simulink model "C28069_LLC_ePWM_V8_230307_PhaeShiftWorking"  (R2022b)
settings: Solver=FixedStepAuto  StartTime=0.0  StopTime=10  RelTol=1e-3  EnableMultiTasking=on
model workspace (MAT data in the model file):
  Comp_DAC = 512
undefined symbols (not defined in the file or in its folder): Down, GPTRIP1SEL, GPTRIP2SEL, PWM_Control, PWM_Gen, PWM_Gen1, SCI_A_Transmit, SCI_A_Transmit_Current_Suffix, SCI_A_Transmit_Duty_Suffix, SCI_A_Transmit_Freq_Suffix, SCI_A_Transmit_OVPFlag_Suffix, SCI_A_Transmit_PFC_Suffix, SCI_A_Transmit_SS_Suffix, SCI_A_Transmit_TBPHS_Suffix, SCI_A_Transmit_VADC_Suffix, SCI_A_Transmit_VAvg_Suffix, SCI_A_Transmit_VBAT_Suffix, SCI_A_Transmit_VBATRef_Suffix, SCI_A_Transmit_Vo_Suffix, TZ1, TZ2, u1, Up
libraries: c2802xlib x92, c280xlib x39, simulink x36, c2000lib x1
(part 14 of 18)

== system C28069_LLC_ePWM_V8_230307_PhaeShiftWorking/Softstart @5kHz/GetADC, FaultProtection, SoftStart  @5KHz/UpdatePWM/Frequency Update ==
  note: For Normal SoftStart
  note: For Reverse SoftStart
  function : TriggerPort  TriggerType=function-call  VariantControl=(inherit)
  Constant : Constant  Value=0  OutDataTypeStr=double
  Constant1 : Constant  Commented=on  Value=0
  Data Store Read : DataStoreRead  Commented=on  DataStoreName=Freq_Value  IndexOptions=Index vector (dialog)  Indices=1  OutputSizes=1
  Data Store Read1 : DataStoreRead  Commented=on  DataStoreName=PFC_OK  IndexOptions=Index vector (dialog)  Indices=1  OutputSizes=1
  Data Store Read10 : DataStoreRead  Commented=on  DataStoreName=OCP_Flag  IndexOptions=Index vector (dialog)  Indices=1  OutputSizes=1
  Data Store Read2 : DataStoreRead  Commented=on  DataStoreName=Duty_Value  IndexOptions=Index vector (dialog)  Indices=1  OutputSizes=1
  Data Store Read3 : DataStoreRead  DataStoreName=Freq_Value  IndexOptions=Index vector (dialog)  Indices=1  OutputSizes=1
  Data Store Read4 : DataStoreRead  DataStoreName=PFC_OK  IndexOptions=Index vector (dialog)  Indices=1  OutputSizes=1
  Data Store Read5 : DataStoreRead  Commented=on  DataStoreName=OVP_Flag  IndexOptions=Index vector (dialog)  Indices=1  OutputSizes=1
  Data Store Read6 : DataStoreRead  DataStoreName=OVP_Flag  IndexOptions=Index vector (dialog)  Indices=1  OutputSizes=1
  Data Store Read7 : DataStoreRead  DataStoreName=Freq_Value_Out  IndexOptions=Index vector (dialog)  Indices=1  OutputSizes=1
  Data Store Read8 : DataStoreRead  Commented=on  DataStoreName=Freq_Value_Out  IndexOptions=Index vector (dialog)  Indices=1  OutputSizes=1
  Data Store Read9 : DataStoreRead  DataStoreName=OCP_Flag  IndexOptions=Index vector (dialog)  Indices=1  OutputSizes=1
  Data Store Write : DataStoreWrite  DataStoreName=Freq_Value_Out  IndexOptions=Index vector (dialog)  Indices=1  OutputSizes=1
  Data Store Write1 : DataStoreWrite  Commented=on  DataStoreName=Freq_Value_Out  IndexOptions=Index vector (dialog)  Indices=1  OutputSizes=1
  Data Type Conversion : DataTypeConversion  Commented=on  OutDataTypeStr=uint16  SaturateOnIntegerOverflow=off  RndMeth=Floor
  Data Type Conversion3 : DataTypeConversion  Commented=on  OutDataTypeStr=uint16  SaturateOnIntegerOverflow=off  RndMeth=Floor
  Data Type Conversion4 : DataTypeConversion  Commented=on  OutDataTypeStr=uint16  SaturateOnIntegerOverflow=off  RndMeth=Floor
  Function Caller : FunctionCaller  Commented=on  FunctionPrototype=PWM_Gen1(u,u1)  InputArgumentSpecifications=<Enter example>  OutputArgumentSpecifications=<Enter example>
  Function Caller1 : FunctionCaller  FunctionPrototype=PWM_Gen(u)  InputArgumentSpecifications=<Enter example>  OutputArgumentSpecifications=<Enter example>
  Product : Product  Commented=on  Inputs=4  OutDataTypeStr=uint16
  Product1 : Product  Inputs=4  OutDataTypeStr=double
  Simulink Function1 : Subsystem  TreatAsAtomicUnit=on
  Simulink Function2 : Subsystem  Commented=on  TreatAsAtomicUnit=on
  Switch : Switch  Criteria=u2 > Threshold  OutDataTypeStr=double  SaturateOnIntegerOverflow=off  InputSameDT=off
  Switch1 : Switch  Commented=on  Criteria=u2 > Threshold  SaturateOnIntegerOverflow=off  InputSameDT=off
  wires:
  Data Store Read8/1 -> Data Type Conversion3/1
  Data Store Read3/1 -> Product1/1
  Data Type Conversion4/1 -> Function Caller/2
  Switch/1 -> Data Store Write/1
  Switch1/1 -> Data Store Write1/1
  Data Store Read6/1 -> Product1/3
  Data Type Conversion3/1 -> Function Caller/1
  Constant/1 -> Switch/3
  Data Store Read9/1 -> Product1/4
  Product/1 -> Switch1/1, Switch1/2
  Data Store Read/1 -> Product/1
  Data Store Read4/1 -> Product1/2
  Constant1/1 -> Switch1/3
  Data Store Read5/1 -> Product/3
  Data Store Read10/1 -> Product/4
  Data Store Read2/1 -> Data Type Conversion4/1
  Product1/1 -> Switch/1, Switch/2
  Data Store Read7/1 -> Function Caller1/1
  Data Type Conversion/1 -> Product/2
  Data Store Read1/1 -> Data Type Conversion/1

== system C28069_LLC_ePWM_V8_230307_PhaeShiftWorking/CloseLoop & Update @ ADCINT, 50kHz/Control/Frequency Update/Simulink Function1/Subsystem1 ==
  Frequency(kHz) : Inport  OutDataTypeStr=double
  Duty(%) : Inport  Port=2
  Constant1 : Constant  Value=90E6
  Divide : Product  Inputs=*/  RndMeth=Zero  SaturateOnIntegerOverflow=on
  Gain : Gain  Gain=1000
  Gain1 : Gain  Gain=1/100
  Gain2 : Gain  Gain=0.5
  Product : Product
  Product1 : Product
  Up-Down Counter : Constant  Value=2
  Out1 : Outport
  Out2 : Outport  Port=2
  Out3 : Outport  Port=3
  wires:
  Up-Down Counter/1 -> Product/2
  Gain/1 -> Product/1
  Product/1 -> Divide/2
  Frequency(kHz)/1 -> Gain/1
  Constant1/1 -> Divide/1
  Divide/1 -> Product1/1, Out1/1
  Duty(%)/1 -> Gain1/1
  Product1/1 -> Out2/1, Gain2/1
  Gain1/1 -> Product1/2
  Gain2/1 -> Out3/1

== system C28069_LLC_ePWM_V8_230307_PhaeShiftWorking/CloseLoop & Update @ ADCINT, 50kHz/Control/Frequency Update/Simulink Function2/Subsystem1 ==
  Frequency(kHz) : Inport
  Duty(%) : Inport  Port=2
  Constant1 : Constant  Value=90E6
  Divide : Product  Inputs=*/  RndMeth=Zero  SaturateOnIntegerOverflow=on
  Gain : Gain  Gain=1000
  Gain1 : Gain  Gain=1/100
  Gain2 : Gain  Gain=0.5
  Product : Product
  Product1 : Product
  Up-Down Counter : Constant  Value=2
  Out1 : Outport
  Out2 : Outport  Port=2
  Out3 : Outport  Port=3
  wires:
  Up-Down Counter/1 -> Product/2
  Gain/1 -> Product/1
  Product/1 -> Divide/2
  Frequency(kHz)/1 -> Gain/1
  Constant1/1 -> Divide/1
  Divide/1 -> Product1/1, Out1/1
  Duty(%)/1 -> Gain1/1
  Product1/1 -> Out2/1, Gain2/1
  Gain1/1 -> Product1/2
  Gain2/1 -> Out3/1

== system C28069_LLC_ePWM_V8_230307_PhaeShiftWorking/CloseLoop & Update @ ADCINT, 50kHz/Control/Frequency Update/Simulink Function3/Subsystem1 ==
  Frequency(kHz) : Inport  OutDataTypeStr=double
  Duty(%) : Inport  Port=2
  Constant1 : Constant  Value=90E6
  Divide : Product  Inputs=*/  RndMeth=Zero  SaturateOnIntegerOverflow=on
  Gain : Gain  Gain=1000
  Gain1 : Gain  Gain=1/100
  Gain2 : Gain  Gain=0.5
  Product : Product
  Product1 : Product
  Up-Down Counter : Constant  Value=2
  Out1 : Outport
  Out2 : Outport  Port=2
  Out3 : Outport  Port=3
  wires:
  Up-Down Counter/1 -> Product/2
  Gain/1 -> Product/1
  Product/1 -> Divide/2
  Frequency(kHz)/1 -> Gain/1
  Constant1/1 -> Divide/1
  Divide/1 -> Product1/1, Out1/1
  Duty(%)/1 -> Gain1/1
  Product1/1 -> Out2/1, Gain2/1
  Gain1/1 -> Product1/2
  Gain2/1 -> Out3/1

== system C28069_LLC_ePWM_V8_230307_PhaeShiftWorking/GetADC, FaultProtection, SoftStart  @5KHz/UpdatePWM/Frequency Update/Simulink Function1/Subsystem1 ==
  Frequency(kHz) : Inport  OutDataTypeStr=double
  Duty(%) : Inport  Port=2
  Constant1 : Constant  Value=90E6
  Divide : Product  Inputs=*/  RndMeth=Zero  SaturateOnIntegerOverflow=on
  Gain : Gain  Gain=1000
  Gain1 : Gain  Gain=1/100
  Gain2 : Gain  Gain=0.5
  Product : Product
  Product1 : Product
  Up-Down Counter : Constant  Value=2
  Out1 : Outport
  Out2 : Outport  Port=2
  Out3 : Outport  Port=3
  wires:
  Gain2/1 -> Out3/1
  Gain1/1 -> Product1/2
  Product1/1 -> Gain2/1, Out2/1
  Duty(%)/1 -> Gain1/1
  Divide/1 -> Out1/1, Product1/1
  Constant1/1 -> Divide/1
  Frequency(kHz)/1 -> Gain/1
  Product/1 -> Divide/2
  Gain/1 -> Product/1
  Up-Down Counter/1 -> Product/2

== system C28069_LLC_ePWM_V8_230307_PhaeShiftWorking/GetADC, FaultProtection, SoftStart  @5KHz/UpdatePWM/Frequency Update/Simulink Function2/Subsystem1 ==
  Frequency(kHz) : Inport
  Duty(%) : Inport  Port=2
  Constant1 : Constant  Value=90E6
  Divide : Product  Inputs=*/  RndMeth=Zero  SaturateOnIntegerOverflow=on
  Gain : Gain  Gain=1000
  Gain1 : Gain  Gain=1/100
  Gain2 : Gain  Gain=0.5
  Product : Product
  Product1 : Product
  Up-Down Counter : Constant  Value=2
  Out1 : Outport
  Out2 : Outport  Port=2
  Out3 : Outport  Port=3
  wires:
  Gain2/1 -> Out3/1
  Gain1/1 -> Product1/2
  Product1/1 -> Gain2/1, Out2/1
  Duty(%)/1 -> Gain1/1
  Divide/1 -> Out1/1, Product1/1
  Constant1/1 -> Divide/1
  Frequency(kHz)/1 -> Gain/1
  Product/1 -> Divide/2
  Gain/1 -> Product/1
  Up-Down Counter/1 -> Product/2

== system C28069_LLC_ePWM_V8_230307_PhaeShiftWorking/GetADC, FaultProtection, SoftStart  @5KHz/UpdatePWM1/Frequency Update/Simulink Function1/Subsystem1 ==
  Frequency(kHz) : Inport  OutDataTypeStr=double
  Duty(%) : Inport  Port=2
  Constant1 : Constant  Value=90E6
  Divide : Product  Inputs=*/  RndMeth=Zero  SaturateOnIntegerOverflow=on
  Gain : Gain  Gain=1000
  Gain1 : Gain  Gain=1/100
  Gain2 : Gain  Gain=0.5
  Product : Product
  Product1 : Product
  Up-Down Counter : Constant  Value=2
  Out1 : Outport
  Out2 : Outport  Port=2
  Out3 : Outport  Port=3
  wires:
  Up-Down Counter/1 -> Product/2
  Gain/1 -> Product/1
  Product/1 -> Divide/2
  Frequency(kHz)/1 -> Gain/1
  Constant1/1 -> Divide/1
  Divide/1 -> Product1/1, Out1/1
  Duty(%)/1 -> Gain1/1
  Product1/1 -> Out2/1, Gain2/1
  Gain1/1 -> Product1/2
  Gain2/1 -> Out3/1

== system C28069_LLC_ePWM_V8_230307_PhaeShiftWorking/GetADC, FaultProtection, SoftStart  @5KHz/UpdatePWM1/Frequency Update/Simulink Function2/Subsystem1 ==
  Frequency(kHz) : Inport
  Duty(%) : Inport  Port=2
  Constant1 : Constant  Value=90E6
  Divide : Product  Inputs=*/  RndMeth=Zero  SaturateOnIntegerOverflow=on
  Gain : Gain  Gain=1000
  Gain1 : Gain  Gain=1/100
  Gain2 : Gain  Gain=0.5
  Product : Product
  Product1 : Product
  Up-Down Counter : Constant  Value=2
  Out1 : Outport
  Out2 : Outport  Port=2
  Out3 : Outport  Port=3
  wires:
  Up-Down Counter/1 -> Product/2
  Gain/1 -> Product/1
  Product/1 -> Divide/2
  Frequency(kHz)/1 -> Gain/1
  Constant1/1 -> Divide/1
  Divide/1 -> Product1/1, Out1/1
  Duty(%)/1 -> Gain1/1
  Product1/1 -> Out2/1, Gain2/1
  Gain1/1 -> Product1/2
  Gain2/1 -> Out3/1

== system C28069_LLC_ePWM_V8_230307_PhaeShiftWorking/GetADC, FaultProtection, SoftStart  @5KHz/UpdatePWM1/Frequency Update/Simulink Function3/Subsystem1 ==
  Frequency(kHz) : Inport  OutDataTypeStr=double
  Duty(%) : Inport  Port=2
  Constant1 : Constant  Value=90E6
  Divide : Product  Inputs=*/  RndMeth=Zero  SaturateOnIntegerOverflow=on
  Gain : Gain  Gain=1000
  Gain1 : Gain  Gain=1/100
  Gain2 : Gain  Gain=0.5
  Product : Product
  Product1 : Product
  Up-Down Counter : Constant  Value=2
  Out1 : Outport
  Out2 : Outport  Port=2
  Out3 : Outport  Port=3
  wires:
  Up-Down Counter/1 -> Product/2
  Gain/1 -> Product/1
  Product/1 -> Divide/2
  Frequency(kHz)/1 -> Gain/1
  Constant1/1 -> Divide/1
  Divide/1 -> Product1/1, Out1/1
  Duty(%)/1 -> Gain1/1
  Product1/1 -> Out2/1, Gain2/1
  Gain1/1 -> Product1/2
  Gain2/1 -> Out3/1

== system C28069_LLC_ePWM_V8_230307_PhaeShiftWorking/GetADC, FaultProtection, SoftStart  @5KHz/UpdatePWM1/SoftStart/If Action Subsystem/ReservseSoftStart1 ==
  function : TriggerPort  TriggerType=function-call  VariantControl=(inherit)
  Chart1 : Stateflow chart  TreatAsAtomicUnit=on
  Constant : Constant  Value=160  OutDataTypeStr=double  SampleTime=Inf
  Constant1 : Constant  Value=200  OutDataTypeStr=double  SampleTime=Inf
  Constant2 : Constant  SampleTime=Inf
  Data Store Read : DataStoreRead  DataStoreName=PFC_OK  IndexOptions=Index vector (dialog)  Indices=1  OutputSizes=1
  Data Store Write1 : DataStoreWrite  DataStoreName=SoftStart_OK_Signal  IndexOptions=Index vector (dialog)  Indices=1  OutputSizes=1
  Data Store Write2 : DataStoreWrite  DataStoreName=Freq_Value  IndexOptions=Index vector (dialog)  Indices=1  OutputSizes=1
  Data Store Write3 : DataStoreWrite  DataStoreName=Duty_Value  IndexOptions=Index vector (dialog)  Indices=1  OutputSizes=1
  Data Type Conversion : DataTypeConversion  OutDataTypeStr=uint16  SaturateOnIntegerOverflow=off  RndMeth=Floor
  Data Type Conversion1 : DataTypeConversion  OutDataTypeStr=uint16  SaturateOnIntegerOverflow=off  RndMeth=Floor
  Data Type Conversion2 : DataTypeConversion  Commented=on  OutDataTypeStr=uint8  SaturateOnIntegerOverflow=off  RndMeth=Floor
  ms : Constant  Commented=on  Value=15  SampleTime=Inf
  wires:
  Constant1/1 -> Chart1/3(Resonant_Frequency)
  Constant/1 -> Chart1/2(Initial_Frequency)
  Data Type Conversion/1 -> Data Store Write2/1
  Chart1/3(Frequency_Adjusted) -> Data Type Conversion/1
  Chart1/1(SoftStart_OK) -> Data Store Write1/1
  Chart1/2(Duty_Adjusted) -> Data Type Conversion1/1
  Data Type Conversion1/1 -> Data Store Write3/1
  Data Store Read/1 -> Chart1/1(PFC_OK)

== system C28069_LLC_ePWM_V8_230307_PhaeShiftWorking/GetADC, FaultProtection, SoftStart  @5KHz/UpdatePWM1/SoftStart/If Action Subsystem/SoftStart1 ==
  function : TriggerPort  TriggerType=function-call  VariantControl=(inherit)
  Chart : Stateflow chart  TreatAsAtomicUnit=on
  Chart1 : Stateflow chart  Commented=on  TreatAsAtomicUnit=on
  Constant : Constant  Commented=on  Value=153  OutDataTypeStr=double  SampleTime=Inf
  Constant1 : Constant  Commented=on  Value=130  OutDataTypeStr=double  SampleTime=Inf
  Constant2 : Constant  Value=15  OutDataTypeStr=double  SampleTime=Inf
  Data Store Read : DataStoreRead  Commented=on  DataStoreName=PFC_OK  IndexOptions=Index vector (dialog)  Indices=1  OutputSizes=1
  Data Store Read1 : DataStoreRead  DataStoreName=PFC_OK  IndexOptions=Index vector (dialog)  Indices=1  OutputSizes=1
  Data Store Read2 : DataStoreRead  DataStoreName=VBAT_Value  IndexOptions=Index vector (dialog)  Indices=1  OutputSizes=1
  Data Store Write : DataStoreWrite  DataStoreName=VBAT_Ref_Value  IndexOptions=Index vector (dialog)  Indices=1  OutputSizes=1
  Data Store Write1 : DataStoreWrite  Commented=on  DataStoreName=SoftStart_OK_Signal  IndexOptions=Index vector (dialog)  Indices=1  OutputSizes=1
  Data Store Write2 : DataStoreWrite  Commented=on  DataStoreName=Freq_Value  IndexOptions=Index vector (dialog)  Indices=1  OutputSizes=1
  Data Store Write3 : DataStoreWrite  DataStoreName=SoftStart_OK_Signal  IndexOptions=Index vector (dialog)  Indices=1  OutputSizes=1
  GPIO21 : c280xlib/Digital Output  GPIO_Number=GPIO16~GPIO23  GPIO_Bit0=off  GPIO_BIT0_Toggle=off  GPIO_Bit1=off  GPIO_BIT1_Toggle=off  GPIO_Bit2=off  GPIO_BIT2_Toggle=off  GPIO_Bit3=off  GPIO_BIT3_Toggle=off  GPIO_Bit4=off  GPIO_BIT4_Toggle=off  GPIO_Bit5=on  GPIO_BIT5_Toggle=off  GPIO_Bit6=off  GPIO_BIT6_Toggle=off  GPIO_Bit7=off  GPIO_BIT7_Toggle=off
  wires:
  Chart1/1(SoftStart_OK) -> Data Store Write1/1
  Chart1/2(Frequency_Adjusted) -> Data Store Write2/1
  Constant/1 -> Chart1/2(Initial_Frequency)
  Constant1/1 -> Chart1/3(Resonant_Frequency)
  Data Store Read/1 -> Chart1/1(PFC_OK)
  Data Store Read1/1 -> GPIO21/1, Chart/1(PFC_OK)
  Constant2/1 -> Chart/3(VBAT_Ref)
  Data Store Read2/1 -> Chart/2(VBAT_Value)
  Chart/1(VBAT_Ref_adjusted) -> Data Store Write/1
  Chart/2(SoftStart_OK) -> Data Store Write3/1

== system C28069_LLC_ePWM_V8_230307_PhaeShiftWorking/Softstart @5kHz/GetADC, FaultProtection, SoftStart  @5KHz/Fault Protection @ 5KHz/If Action Subsystem/OCP ==
  note: 1900 = @>1.9A Load will trigger
  note: False
  note: Average the value
  note: True
  function : TriggerPort  TriggerType=function-call  VariantControl=(inherit)
  ADC : c2802xlib/ADC  Commented=on  blkParamProc=C2000  ADCModule=1  samplingMode=Single sample mode  ADCResolution=12-bit (Single-ended input)  useSOC1=SOC0  useSOC2=SOC0_SOC1  SOCAcquisitionWindow=7  SOCTriggerSource=ePWM5_ADCSOCA  SOCInterruptTrigger=No ADCINT  Ts=-1  dType=uint16  postInterrupt=off  interruptSel=ADCINT1  ADCINTContinuous=off  endma=off  chdma=1  conv1=ADCINA2  conv2=ADCINA0 and ADCINB0  conv1_Type4=ADCIN0  conv2_Type4=ADCIN0 and ADCIN1
      settings: LibrarySourceBlock=c2806xlib/ADC
  Constant3 : Constant  Value=0  OutDataTypeStr=single
  Data Store Read : DataStoreRead  DataStoreName=OCP_Flag  IndexOptions=Index vector (dialog)  Indices=1  OutputSizes=1
  Data Store Read1 : DataStoreRead  DataStoreName=IoutCurrentBAT_Value  IndexOptions=Index vector (dialog)  Indices=1  OutputSizes=1
  Data Store Write2 : DataStoreWrite  DataStoreName=OCP_Flag  IndexOptions=Index vector (dialog)  Indices=1  OutputSizes=1
  Data Type Conversion1 : DataTypeConversion  OutDataTypeStr=double  SaturateOnIntegerOverflow=off  RndMeth=Floor
  Delay : Delay  Commented=on  DelayLength=1
  Delay1 : Delay  Commented=on
  Delay2 : Delay  Commented=on  DelayLength=3
  Delay3 : Delay  Commented=on  DelayLength=4
  Delay4 : Delay  Commented=on  DelayLength=5
  Display7 : Display
  Gain : Gain  Commented=on  Gain=1/6  OutDataTypeStr=uint16
  Sum : Sum  Commented=on  Inputs=|++++++
  Switch : Switch  Criteria=u2 > Threshold  Threshold=2100  OutDataTypeStr=single  SaturateOnIntegerOverflow=off  InputSameDT=off
  wires:
  Data Store Read1/1 -> Switch/2, Display7/1
  Delay4/1 -> Sum/6
  Delay3/1 -> Sum/5
  Gain/1 -> Delay/1, Delay1/1, Delay2/1, Delay3/1, Delay4/1
  Delay/1 -> Sum/2
  Delay1/1 -> Sum/3
  Delay2/1 -> Sum/4
  Sum/1 -> Gain/1
  Data Type Conversion1/1 -> Data Store Write2/1
  Data Store Read/1 -> Switch/3
  Constant3/1 -> Switch/1
  Switch/1 -> Data Type Conversion1/1
  ADC/1 -> Sum/1

== system C28069_LLC_ePWM_V8_230307_PhaeShiftWorking/Softstart @5kHz/GetADC, FaultProtection, SoftStart  @5KHz/Fault Protection @ 5KHz/If Action Subsystem/OVP ==
  note: True
  note: Average the value
  note: False
  note: >92Vdc will trigger
  function : TriggerPort  TriggerType=function-call  VariantControl=(inherit)
  ADC : c2802xlib/ADC  Commented=on  blkParamProc=C2000  ADCModule=1  samplingMode=Single sample mode  ADCResolution=12-bit (Single-ended input)  useSOC1=SOC0  useSOC2=SOC0_SOC1  SOCAcquisitionWindow=7  SOCTriggerSource=ePWM5_ADCSOCA  SOCInterruptTrigger=No ADCINT  Ts=-1  dType=uint16  postInterrupt=off  interruptSel=ADCINT1  ADCINTContinuous=off  endma=off  chdma=1  conv1=ADCINA2  conv2=ADCINA0 and ADCINB0  conv1_Type4=ADCIN0  conv2_Type4=ADCIN0 and ADCIN1
      settings: LibrarySourceBlock=c2806xlib/ADC
  Constant3 : Constant  Value=0  OutDataTypeStr=single
  Data Store Read : DataStoreRead  DataStoreName=OVP_Flag  IndexOptions=Index vector (dialog)  Indices=1  OutputSizes=1
  Data Store Read1 : DataStoreRead  DataStoreName=VBAT_Value  IndexOptions=Index vector (dialog)  Indices=1  OutputSizes=1
  Data Store Write2 : DataStoreWrite  DataStoreName=OVP_Flag  IndexOptions=Index vector (dialog)  Indices=1  OutputSizes=1
  Data Type Conversion1 : DataTypeConversion  OutDataTypeStr=double  SaturateOnIntegerOverflow=off  RndMeth=Floor
  Delay : Delay  Commented=on  DelayLength=1
  Delay1 : Delay  Commented=on
  Delay2 : Delay  Commented=on  DelayLength=3
  Delay3 : Delay  Commented=on  DelayLength=4
  Delay4 : Delay  Commented=on  DelayLength=5
  Display7 : Display
  Gain : Gain  Commented=on  Gain=1/6  OutDataTypeStr=uint16
  Sum : Sum  Commented=on  Inputs=|++++++
  Switch : Switch  Criteria=u2 > Threshold  Threshold=35  OutDataTypeStr=single  SaturateOnIntegerOverflow=off  InputSameDT=off
  wires:
  ADC/1 -> Sum/1
  Switch/1 -> Data Type Conversion1/1
  Constant3/1 -> Switch/1
  Data Store Read/1 -> Switch/3
  Data Type Conversion1/1 -> Data Store Write2/1
  Sum/1 -> Gain/1
  Delay2/1 -> Sum/4
  Delay1/1 -> Sum/3
  Delay/1 -> Sum/2
  Gain/1 -> Delay4/1, Delay3/1, Delay2/1, Delay1/1, Delay/1
  Delay3/1 -> Sum/5
  Delay4/1 -> Sum/6
  Data Store Read1/1 -> Display7/1, Switch/2

== system C28069_LLC_ePWM_V8_230307_PhaeShiftWorking/Softstart @5kHz/GetADC, FaultProtection, SoftStart  @5KHz/Fault Protection @ 5KHz/If Action Subsystem/TestToCheckOVPFlag ==
  note: Comment out GPIO14 when flash to MB, as SCI_B using GPIO14
  note: Test to check if this OVP_Flag is working
  function : TriggerPort  TriggerType=function-call  VariantControl=(inherit)
  Data Store Read : DataStoreRead  DataStoreName=OVP_Flag  IndexOptions=Index vector (dialog)  Indices=1  OutputSizes=1
  GPIO14 Test : c280xlib/Digital Output  GPIO_Number=GPIO8~GPIO15  GPIO_Bit0=off  GPIO_BIT0_Toggle=off  GPIO_Bit1=off  GPIO_BIT1_Toggle=off  GPIO_Bit2=off  GPIO_BIT2_Toggle=off  GPIO_Bit3=off  GPIO_BIT3_Toggle=off  GPIO_Bit4=off  GPIO_BIT4_Toggle=off  GPIO_Bit5=off  GPIO_BIT5_Toggle=off  GPIO_Bit6=on  GPIO_BIT6_Toggle=off  GPIO_Bit7=off  GPIO_BIT7_Toggle=off
  wires:
  Data Store Read/1 -> GPIO14 Test/1

== system C28069_LLC_ePWM_V8_230307_PhaeShiftWorking/Softstart @5kHz/GetADC, FaultProtection, SoftStart  @5KHz/Fault Protection @ 5KHz1/If Action Subsystem/OCP ==
  note: 1900 = @>1.9A Load will trigger
  note: False
  note: Average the value
  note: True
  function : TriggerPort  TriggerType=function-call  VariantControl=(inherit)
  ADC : c2802xlib/ADC  Commented=on  blkParamProc=C2000  ADCModule=1  samplingMode=Single sample mode  ADCResolution=12-bit (Single-ended input)  useSOC1=SOC0  useSOC2=SOC0_SOC1  SOCAcquisitionWindow=7  SOCTriggerSource=ePWM5_ADCSOCA  SOCInterruptTrigger=No ADCINT  Ts=-1  dType=uint16  postInterrupt=off  interruptSel=ADCINT1  ADCINTContinuous=off  endma=off  chdma=1  conv1=ADCINA2  conv2=ADCINA0 and ADCINB0  conv1_Type4=ADCIN0  conv2_Type4=ADCIN0 and ADCIN1
      settings: LibrarySourceBlock=c2806xlib/ADC
  Constant3 : Constant  Value=0  OutDataTypeStr=single
  Data Store Read : DataStoreRead  DataStoreName=OCP_Flag  IndexOptions=Index vector (dialog)  Indices=1  OutputSizes=1
  Data Store Read1 : DataStoreRead  DataStoreName=IoutCurrentBAT_Value  IndexOptions=Index vector (dialog)  Indices=1  OutputSizes=1
  Data Store Write2 : DataStoreWrite  DataStoreName=OCP_Flag  IndexOptions=Index vector (dialog)  Indices=1  OutputSizes=1
  Data Type Conversion1 : DataTypeConversion  OutDataTypeStr=double  SaturateOnIntegerOverflow=off  RndMeth=Floor
  Delay : Delay  Commented=on  DelayLength=1
  Delay1 : Delay  Commented=on
  Delay2 : Delay  Commented=on  DelayLength=3
  Delay3 : Delay  Commented=on  DelayLength=4
  Delay4 : Delay  Commented=on  DelayLength=5
  Display7 : Display
  Gain : Gain  Commented=on  Gain=1/6  OutDataTypeStr=uint16
  Sum : Sum  Commented=on  Inputs=|++++++
  Switch : Switch  Criteria=u2 > Threshold  Threshold=2100  OutDataTypeStr=single  SaturateOnIntegerOverflow=off  InputSameDT=off
  wires:
  Data Store Read1/1 -> Switch/2, Display7/1
  Delay4/1 -> Sum/6
  Delay3/1 -> Sum/5
  Gain/1 -> Delay/1, Delay1/1, Delay2/1, Delay3/1, Delay4/1
  Delay/1 -> Sum/2
  Delay1/1 -> Sum/3
  Delay2/1 -> Sum/4
  Sum/1 -> Gain/1
  Data Type Conversion1/1 -> Data Store Write2/1
  Data Store Read/1 -> Switch/3
  Constant3/1 -> Switch/1
  Switch/1 -> Data Type Conversion1/1
  ADC/1 -> Sum/1

== system C28069_LLC_ePWM_V8_230307_PhaeShiftWorking/Softstart @5kHz/GetADC, FaultProtection, SoftStart  @5KHz/Fault Protection @ 5KHz1/If Action Subsystem/OVP ==
  note: True
  note: Average the value
  note: False
  note: >92Vdc will trigger
  function : TriggerPort  TriggerType=function-call  VariantControl=(inherit)
  ADC : c2802xlib/ADC  Commented=on  blkParamProc=C2000  ADCModule=1  samplingMode=Single sample mode  ADCResolution=12-bit (Single-ended input)  useSOC1=SOC0  useSOC2=SOC0_SOC1  SOCAcquisitionWindow=7  SOCTriggerSource=ePWM5_ADCSOCA  SOCInterruptTrigger=No ADCINT  Ts=-1  dType=uint16  postInterrupt=off  interruptSel=ADCINT1  ADCINTContinuous=off  endma=off  chdma=1  conv1=ADCINA2  conv2=ADCINA0 and ADCINB0  conv1_Type4=ADCIN0  conv2_Type4=ADCIN0 and ADCIN1
      settings: LibrarySourceBlock=c2806xlib/ADC
  Constant3 : Constant  Value=0  OutDataTypeStr=single
  Data Store Read : DataStoreRead  DataStoreName=OVP_Flag  IndexOptions=Index vector (dialog)  Indices=1  OutputSizes=1
  Data Store Read1 : DataStoreRead  DataStoreName=VBAT_Value  IndexOptions=Index vector (dialog)  Indices=1  OutputSizes=1
  Data Store Write2 : DataStoreWrite  DataStoreName=OVP_Flag  IndexOptions=Index vector (dialog)  Indices=1  OutputSizes=1
  Data Type Conversion1 : DataTypeConversion  OutDataTypeStr=double  SaturateOnIntegerOverflow=off  RndMeth=Floor
  Delay : Delay  Commented=on  DelayLength=1
  Delay1 : Delay  Commented=on
  Delay2 : Delay  Commented=on  DelayLength=3
  Delay3 : Delay  Commented=on  DelayLength=4
  Delay4 : Delay  Commented=on  DelayLength=5
  Display7 : Display
  Gain : Gain  Commented=on  Gain=1/6  OutDataTypeStr=uint16
  Sum : Sum  Commented=on  Inputs=|++++++
  Switch : Switch  Criteria=u2 > Threshold  Threshold=35  OutDataTypeStr=single  SaturateOnIntegerOverflow=off  InputSameDT=off
  wires:
  ADC/1 -> Sum/1
  Switch/1 -> Data Type Conversion1/1
  Constant3/1 -> Switch/1
  Data Store Read/1 -> Switch/3
  Data Type Conversion1/1 -> Data Store Write2/1
  Sum/1 -> Gain/1
  Delay2/1 -> Sum/4
  Delay1/1 -> Sum/3
  Delay/1 -> Sum/2
  Gain/1 -> Delay4/1, Delay3/1, Delay2/1, Delay1/1, Delay/1
  Delay3/1 -> Sum/5
  Delay4/1 -> Sum/6
  Data Store Read1/1 -> Display7/1, Switch/2

== system C28069_LLC_ePWM_V8_230307_PhaeShiftWorking/Softstart @5kHz/GetADC, FaultProtection, SoftStart  @5KHz/Fault Protection @ 5KHz1/If Action Subsystem/TestToCheckOVPFlag ==
  note: Comment out GPIO14 when flash to MB, as SCI_B using GPIO14
  note: Test to check if this OVP_Flag is working
  function : TriggerPort  TriggerType=function-call  VariantControl=(inherit)
  Data Store Read : DataStoreRead  DataStoreName=OVP_Flag  IndexOptions=Index vector (dialog)  Indices=1  OutputSizes=1
  GPIO14 Test : c280xlib/Digital Output  GPIO_Number=GPIO8~GPIO15  GPIO_Bit0=off  GPIO_BIT0_Toggle=off  GPIO_Bit1=off  GPIO_BIT1_Toggle=off  GPIO_Bit2=off  GPIO_BIT2_Toggle=off  GPIO_Bit3=off  GPIO_BIT3_Toggle=off  GPIO_Bit4=off  GPIO_BIT4_Toggle=off  GPIO_Bit5=off  GPIO_BIT5_Toggle=off  GPIO_Bit6=on  GPIO_BIT6_Toggle=off  GPIO_Bit7=off  GPIO_BIT7_Toggle=off
  wires:
  Data Store Read/1 -> GPIO14 Test/1

== system C28069_LLC_ePWM_V8_230307_PhaeShiftWorking/Softstart @5kHz/GetADC, FaultProtection, SoftStart  @5KHz/Frequency Update/Simulink Function1/Subsystem1 ==
  Frequency(kHz) : Inport  OutDataTypeStr=double
  Duty(%) : Inport  Port=2
  Constant1 : Constant  Value=90E6
  Divide : Product  Inputs=*/  RndMeth=Zero  SaturateOnIntegerOverflow=on
  Gain : Gain  Gain=1000
  Gain1 : Gain  Gain=1/100
  Gain2 : Gain  Gain=0.5
  Product : Product
  Product1 : Product
  Up-Down Counter : Constant  Value=2
  Out1 : Outport
  Out2 : Outport  Port=2
  Out3 : Outport  Port=3
  wires:
  Up-Down Counter/1 -> Product/2
  Gain/1 -> Product/1
  Product/1 -> Divide/2
  Frequency(kHz)/1 -> Gain/1
  Constant1/1 -> Divide/1
  Divide/1 -> Product1/1, Out1/1
  Duty(%)/1 -> Gain1/1
  Product1/1 -> Out2/1, Gain2/1
  Gain1/1 -> Product1/2
  Gain2/1 -> Out3/1

== system C28069_LLC_ePWM_V8_230307_PhaeShiftWorking/Softstart @5kHz/GetADC, FaultProtection, SoftStart  @5KHz/Frequency Update/Simulink Function2/Subsystem1 ==
  Frequency(kHz) : Inport
  Duty(%) : Inport  Port=2
  Constant1 : Constant  Value=90E6
  Divide : Product  Inputs=*/  RndMeth=Zero  SaturateOnIntegerOverflow=on
  Gain : Gain  Gain=1000
  Gain1 : Gain  Gain=1/100
  Gain2 : Gain  Gain=0.5
  Product : Product
  Product1 : Product
  Up-Down Counter : Constant  Value=2
  Out1 : Outport
  Out2 : Outport  Port=2
  Out3 : Outport  Port=3
  wires:
  Up-Down Counter/1 -> Product/2
  Gain/1 -> Product/1
  Product/1 -> Divide/2
  Frequency(kHz)/1 -> Gain/1
  Constant1/1 -> Divide/1
  Divide/1 -> Product1/1, Out1/1
  Duty(%)/1 -> Gain1/1
  Product1/1 -> Out2/1, Gain2/1
  Gain1/1 -> Product1/2
  Gain2/1 -> Out3/1

== system C28069_LLC_ePWM_V8_230307_PhaeShiftWorking/Softstart @5kHz/GetADC, FaultProtection, SoftStart  @5KHz/Frequency Update/Simulink Function3/Subsystem1 ==
  Frequency(kHz) : Inport  OutDataTypeStr=double
  Duty(%) : Inport  Port=2
  Constant1 : Constant  Value=90E6
  Divide : Product  Inputs=*/  RndMeth=Zero  SaturateOnIntegerOverflow=on
  Gain : Gain  Gain=1000
  Gain1 : Gain  Gain=1/100
  Gain2 : Gain  Gain=0.5
  Product : Product
  Product1 : Product
  Up-Down Counter : Constant  Value=2
  Out1 : Outport
  Out2 : Outport  Port=2
  Out3 : Outport  Port=3
  wires:
  Up-Down Counter/1 -> Product/2
  Gain/1 -> Product/1
  Product/1 -> Divide/2
  Frequency(kHz)/1 -> Gain/1
  Constant1/1 -> Divide/1
  Divide/1 -> Product1/1, Out1/1
  Duty(%)/1 -> Gain1/1
  Product1/1 -> Out2/1, Gain2/1
  Gain1/1 -> Product1/2
  Gain2/1 -> Out3/1

== system C28069_LLC_ePWM_V8_230307_PhaeShiftWorking/Softstart @5kHz/GetADC, FaultProtection, SoftStart  @5KHz/SoftStart/If Action Subsystem/ReservseSoftStart ==
  function : TriggerPort  TriggerType=function-call  VariantControl=(inherit)
  Chart1 : Stateflow chart  TreatAsAtomicUnit=on
  Constant : Constant  Value=160  OutDataTypeStr=double  SampleTime=Inf
  Constant1 : Constant  Value=200  OutDataTypeStr=double  SampleTime=Inf
  Constant2 : Constant  SampleTime=Inf
  Data Store Read : DataStoreRead  DataStoreName=PFC_OK  IndexOptions=Index vector (dialog)  Indices=1  OutputSizes=1
  Data Store Write1 : DataStoreWrite  DataStoreName=SoftStart_OK_Signal  IndexOptions=Index vector (dialog)  Indices=1  OutputSizes=1
  Data Store Write2 : DataStoreWrite  DataStoreName=Freq_Value  IndexOptions=Index vector (dialog)  Indices=1  OutputSizes=1
  Data Store Write3 : DataStoreWrite  DataStoreName=Duty_Value  IndexOptions=Index vector (dialog)  Indices=1  OutputSizes=1
  Data Type Conversion : DataTypeConversion  OutDataTypeStr=uint16  SaturateOnIntegerOverflow=off  RndMeth=Floor
  Data Type Conversion1 : DataTypeConversion  OutDataTypeStr=uint16  SaturateOnIntegerOverflow=off  RndMeth=Floor
  Data Type Conversion2 : DataTypeConversion  Commented=on  OutDataTypeStr=uint8  SaturateOnIntegerOverflow=off  RndMeth=Floor
  ms : Constant  Commented=on  Value=15  SampleTime=Inf
  wires:
  Constant1/1 -> Chart1/3(Resonant_Frequency)
  Constant/1 -> Chart1/2(Initial_Frequency)
  Data Type Conversion/1 -> Data Store Write2/1
  Chart1/3(Frequency_Adjusted) -> Data Type Conversion/1
  Chart1/1(SoftStart_OK) -> Data Store Write1/1
  Chart1/2(Duty_Adjusted) -> Data Type Conversion1/1
  Data Type Conversion1/1 -> Data Store Write3/1
  Data Store Read/1 -> Chart1/1(PFC_OK)

== system C28069_LLC_ePWM_V8_230307_PhaeShiftWorking/Softstart @5kHz/GetADC, FaultProtection, SoftStart  @5KHz/SoftStart/If Action Subsystem/SoftStart ==
  function : TriggerPort  TriggerType=function-call  VariantControl=(inherit)
  Chart1 : Stateflow chart  TreatAsAtomicUnit=on
  Constant : Constant  Value=153  OutDataTypeStr=double  SampleTime=Inf
  Constant1 : Constant  Value=130  OutDataTypeStr=double  SampleTime=Inf
  Data Store Read : DataStoreRead  DataStoreName=PFC_OK  IndexOptions=Index vector (dialog)  Indices=1  OutputSizes=1
  Data Store Write1 : DataStoreWrite  DataStoreName=SoftStart_OK_Signal  IndexOptions=Index vector (dialog)  Indices=1  OutputSizes=1
  Data Store Write2 : DataStoreWrite  DataStoreName=Freq_Value  IndexOptions=Index vector (dialog)  Indices=1  OutputSizes=1
  wires:
  Chart1/1(SoftStart_OK) -> Data Store Write1/1
  Chart1/2(Frequency_Adjusted) -> Data Store Write2/1
  Constant/1 -> Chart1/2(Initial_Frequency)
  Constant1/1 -> Chart1/3(Resonant_Frequency)
  Data Store Read/1 -> Chart1/1(PFC_OK)

== system C28069_LLC_ePWM_V8_230307_PhaeShiftWorking/Softstart @5kHz/GetADC, FaultProtection, SoftStart  @5KHz/SoftStart1/If Action Subsystem/ReservseSoftStart1 ==
  function : TriggerPort  TriggerType=function-call  VariantControl=(inherit)
  Chart1 : Stateflow chart  TreatAsAtomicUnit=on
  Constant : Constant  Value=160  OutDataTypeStr=double  SampleTime=Inf
  Constant1 : Constant  Value=200  OutDataTypeStr=double  SampleTime=Inf
  Constant2 : Constant  SampleTime=Inf
  Data Store Read : DataStoreRead  DataStoreName=PFC_OK  IndexOptions=Index vector (dialog)  Indices=1  OutputSizes=1
  Data Store Write1 : DataStoreWrite  DataStoreName=SoftStart_OK_Signal  IndexOptions=Index vector (dialog)  Indices=1  OutputSizes=1
  Data Store Write2 : DataStoreWrite  DataStoreName=Freq_Value  IndexOptions=Index vector (dialog)  Indices=1  OutputSizes=1
  Data Store Write3 : DataStoreWrite  DataStoreName=Duty_Value  IndexOptions=Index vector (dialog)  Indices=1  OutputSizes=1
  Data Type Conversion : DataTypeConversion  OutDataTypeStr=uint16  SaturateOnIntegerOverflow=off  RndMeth=Floor
  Data Type Conversion1 : DataTypeConversion  OutDataTypeStr=uint16  SaturateOnIntegerOverflow=off  RndMeth=Floor
  Data Type Conversion2 : DataTypeConversion  Commented=on  OutDataTypeStr=uint8  SaturateOnIntegerOverflow=off  RndMeth=Floor
  ms : Constant  Commented=on  Value=15  SampleTime=Inf
  wires:
  Constant1/1 -> Chart1/3(Resonant_Frequency)
  Constant/1 -> Chart1/2(Initial_Frequency)
  Data Type Conversion/1 -> Data Store Write2/1
  Chart1/3(Frequency_Adjusted) -> Data Type Conversion/1
  Chart1/1(SoftStart_OK) -> Data Store Write1/1
  Chart1/2(Duty_Adjusted) -> Data Type Conversion1/1
  Data Type Conversion1/1 -> Data Store Write3/1
  Data Store Read/1 -> Chart1/1(PFC_OK)

== system C28069_LLC_ePWM_V8_230307_PhaeShiftWorking/Softstart @5kHz/GetADC, FaultProtection, SoftStart  @5KHz/SoftStart1/If Action Subsystem/SoftStart1 ==
  function : TriggerPort  TriggerType=function-call  VariantControl=(inherit)
  Chart : Stateflow chart  TreatAsAtomicUnit=on
  Chart1 : Stateflow chart  Commented=on  TreatAsAtomicUnit=on
  Constant : Constant  Commented=on  Value=153  OutDataTypeStr=double  SampleTime=Inf
  Constant1 : Constant  Commented=on  Value=130  OutDataTypeStr=double  SampleTime=Inf
  Constant2 : Constant  OutDataTypeStr=double  SampleTime=Inf
  Data Store Read : DataStoreRead  Commented=on  DataStoreName=PFC_OK  IndexOptions=Index vector (dialog)  Indices=1  OutputSizes=1
  Data Store Read1 : DataStoreRead  DataStoreName=PFC_OK  IndexOptions=Index vector (dialog)  Indices=1  OutputSizes=1
  Data Store Read2 : DataStoreRead  DataStoreName=VBAT_Value  IndexOptions=Index vector (dialog)  Indices=1  OutputSizes=1
  Data Store Write : DataStoreWrite  DataStoreName=VBAT_Ref_Value  IndexOptions=Index vector (dialog)  Indices=1  OutputSizes=1
  Data Store Write1 : DataStoreWrite  Commented=on  DataStoreName=SoftStart_OK_Signal  IndexOptions=Index vector (dialog)  Indices=1  OutputSizes=1
  Data Store Write2 : DataStoreWrite  Commented=on  DataStoreName=Freq_Value  IndexOptions=Index vector (dialog)  Indices=1  OutputSizes=1
  Data Store Write3 : DataStoreWrite  DataStoreName=SoftStart_OK_Signal  IndexOptions=Index vector (dialog)  Indices=1  OutputSizes=1
  wires:
  Chart1/1(SoftStart_OK) -> Data Store Write1/1
  Chart1/2(Frequency_Adjusted) -> Data Store Write2/1
  Constant/1 -> Chart1/2(Initial_Frequency)
  Constant1/1 -> Chart1/3(Resonant_Frequency)
  Data Store Read/1 -> Chart1/1(PFC_OK)
  Data Store Read1/1 -> Chart/1(PFC_OK)
  Constant2/1 -> Chart/3(VBAT_Ref)
  Data Store Read2/1 -> Chart/2(VBAT_Value)
  Chart/1(VBAT_Ref_adjusted) -> Data Store Write/1
  Chart/2(SoftStart_OK) -> Data Store Write3/1

== system C28069_LLC_ePWM_V8_230307_PhaeShiftWorking/Softstart @5kHz/GetADC, FaultProtection, SoftStart  @5KHz/UpdatePWM/Close Loop Regulation/If Action Subsystem ==
  note: Take note : All of them are ADC values.
  note: Voltage regulation for LLC (Not done yet)
  note: Regulation the Output Voltage and Sweeping the frequency accordingly to meet the output voltage.
      | Than if hit the 'max' frequency, it will trigger to reduce the duty cycle.
  Action Port : ActionPort
  Chart : Stateflow chart  TreatAsAtomicUnit=on
  Constant70 : Constant  Value=100  OutDataTypeStr=double
  Constant71 : Constant  Value=180  OutDataTypeStr=double
  Data Store Read : DataStoreRead  DataStoreName=VBAT_Value  IndexOptions=Index vector (dialog)  Indices=1  OutputSizes=1
  Data Store Read1 : DataStoreRead  DataStoreName=Freq_Value  IndexOptions=Index vector (dialog)  Indices=1  OutputSizes=1
  Data Store Write1 : DataStoreWrite  DataStoreName=Freq_Value  IndexOptions=Index vector (dialog)  Indices=1  OutputSizes=1
  Data Type Conversion : DataTypeConversion  OutDataTypeStr=double  SaturateOnIntegerOverflow=off  RndMeth=Floor
  Saturation Dynamic1 : simulink/Discontinuities/Saturation Dynamic  OutMin=[]  OutMax=[]  OutDataTypeStr=double  OutputDataTypeScalingMode=single  OutDataType=single  OutScaling=2^-10  DoSatur=off
  Testing30Vout ReferencePoint : Constant  Value=25  OutDataTypeStr=double
  V_err : Sum  Inputs=|+-  AccumDataTypeStr=double  OutDataTypeStr=double
  wires:
  Constant71/1 -> [Max_Freq]
  Testing30Vout ReferencePoint/1 -> V_err/1
  Data Store Read/1 -> Data Type Conversion/1
  Saturation Dynamic1/1 -> Data Store Write1/1
  V_err/1 -> Chart/1(input_u)
  [Max_Freq] -> Saturation Dynamic1/1
  [Min_Freq] -> Saturation Dynamic1/3
  Chart/1(output_y) -> Saturation Dynamic1/2
  Constant70/1 -> [Min_Freq]
  Data Store Read1/1 -> Chart/2(prev_freq)
  Data Type Conversion/1 -> V_err/2
